simulink model "washingmachine"  (R2024b)
settings: Solver=VariableStepAuto  StartTime=0.0  StopTime=120  RelTol=1e-3
settings Model: Creator=Kumaresh Raj  LastModifiedBy=Kumaresh Raj

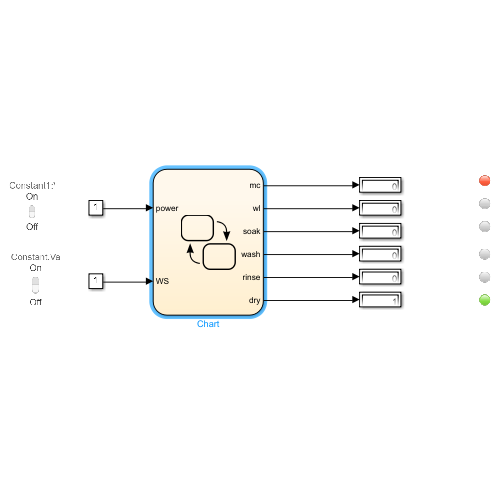
[thumbnail: Simulink's stored preview of the top-level diagram]
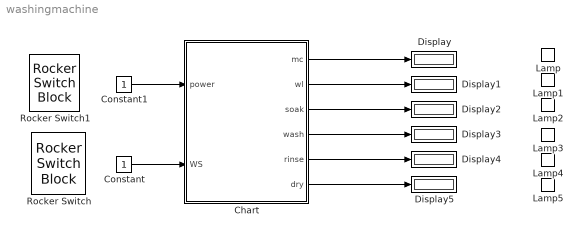
== system washingmachine ==
  Chart : Stateflow chart  TreatAsAtomicUnit=on
  Constant : Constant
  Constant1 : Constant
  Display{,1..5} (6 alike) : Display
  Lamp{,1..5} (6 alike) : LampBlock  LabelPosition=Hide
  Rocker Switch : RockerSwitchBlock
      settings: Values={{'Off', 'On'}, [0 1]}
  Rocker Switch1 : RockerSwitchBlock
      settings: Values={{'Off', 'On'}, [0 1]}
  wires:
  Constant/1 -> Chart/2(WS)
  Constant1/1 -> Chart/1(power)
  Chart/1(mc) -> Display/1
  Chart/2(wl) -> Display1/1
  Chart/3(soak) -> Display2/1
  Chart/4(wash) -> Display3/1
  Chart/5(rinse) -> Display4/1
  Chart/6(dry) -> Display5/1

== stateflow chart washingmachine/Chart ==
  state OFF
    entry:
    mc=0;
  state ON
    entry:
    mc=1;
  state low
    entry:
    wl=0;
  state waterlevelcheck
  state high
    entry:
    wl=1;
  state SOAKING
    entry:
    soak=1;
    during:
    wl=0;
  state WASHING
    entry:
    wash=1;
    during:
    soak=0;
  state RINSING
    entry:
    rinse=1;
    during:
    wash=0;
  state DRYING
    entry:
    dry=1;
    during:
    rinse=0;
  (default) -> OFF
  OFF -> ON : [power==1]
  DRYING -> OFF : after(10,sec)
  ON -> OFF [order 1] : [power==0]
  low -> OFF
  ON -> waterlevelcheck [order 2]
  waterlevelcheck -> low [order 1] : [WS==0]
  waterlevelcheck -> high [order 2] : [WS==1]
  high -> SOAKING : after(5,sec)
  SOAKING -> WASHING : after(25,sec)
  WASHING -> RINSING : after(50,sec)
  RINSING -> DRYING : after(15,sec)
  data: mc output; wl output; soak output; wash output; rinse output; dry output; power input; WS input
